simulink model "example_F41"  (R2016b)
settings: Solver=ode15s  StartTime=0.0  StopTime=50.00  RelTol=1e-3
PreLoadFcn:
  | R = 0.3;
  | L = 1e-6;
  | J = 6;
  | K = 0.5;
  | k = 0.5;
settings Model: Creator=training-ah  LastModifiedBy=training-ah

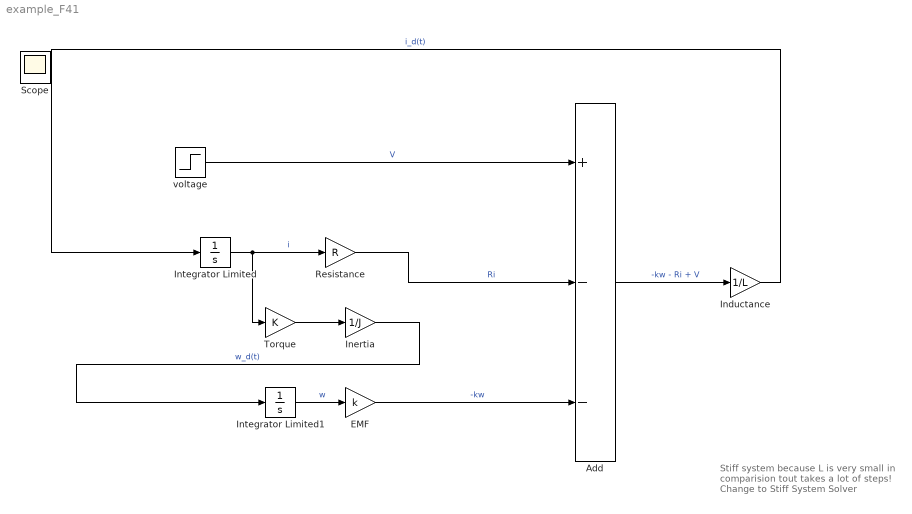
== system example_F41 ==
  note: Stiff system because L is very small in
      | comparision
      | tout takes a lot of steps!
      | Change to Stiff System Solver
  Add : Sum  Inputs=+--
  EMF : Gain  Gain=k
  Inductance : Gain  Gain=1/L
  Inertia : Gain  Gain=1/J
  Integrator Limited : Integrator  UpperSaturationLimit=1  LowerSaturationLimit=0
  Integrator Limited1 : Integrator  UpperSaturationLimit=1  LowerSaturationLimit=0
  Resistance : Gain  Gain=R
  Torque : Gain  Gain=K
  voltage : Step  SampleTime=0
  Scope : Scope
  wires:
  Inductance/1 -> Integrator Limited/1  "i_d(t)"
  Integrator Limited/1 -> Torque/1, Resistance/1  "i"
  voltage/1 -> Add/1  "V"
  Resistance/1 -> Add/2  "Ri"
  EMF/1 -> Add/3  "-kw"
  Inertia/1 -> Integrator Limited1/1  "w_d(t)"
  Integrator Limited1/1 -> EMF/1  "w"
  Add/1 -> Inductance/1  "-kw - Ri + V"
  Torque/1 -> Inertia/1
